simulink model "generator_mode"  (Simulink 7.1)
settings: Solver=ode45  StartTime=0.0  StopTime=10.0  RelTol=1e-3
undefined symbols (not defined in the file or in its folder): fcn
settings Model: Creator=lv  LastModifiedBy=lv

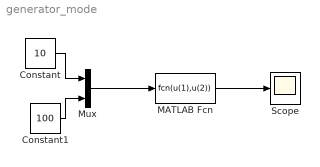
== system generator_mode ==
  Constant : Constant  Value=10  OutDataType=sfix(16)  OutScaling=2^0
  Constant1 : Constant  Value=100  OutDataType=sfix(16)  OutScaling=2^0
  MATLAB Fcn : MATLABFcn  MATLABFcn=fcn(u(1),u(2))
  Mux : Mux  Inputs=2
  Scope : Scope
  wires:
  Mux/1 -> MATLAB Fcn/1
  Constant/1 -> Mux/1
  Constant1/1 -> Mux/2
  MATLAB Fcn/1 -> Scope/1
